simulink model "DYC0928"  (R2022b)
settings: Solver=VariableStepAuto  StartTime=0.0  StopTime=40  RelTol=1e-3
values from neighbouring files (symbols this model uses):
  Caf = 460    [trqvparameter.m]
  Car = 440    [trqvparameter.m]
  dwf = 1.2    [trqvparameter.m]
  dwr = 1.2    [trqvparameter.m]
  h = 0.29    [trqvparameter.m]
  i1 = 11.4    [trqvparameter.m]
  i2 = 3.4    [trqvparameter.m]
  Iz = 105    [trqvparameter.m]
  Kc = 10    [trqvparameter.m]
  Ki = 20    [trqvparameter.m]
  Kp = 30    [trqvparameter.m]
  lf = 0.761    [trqvparameter.m]
  lr = 0.831    [trqvparameter.m]
  m = 340    [trqvparameter.m]
  Rt = 0.2    [trqvparameter.m]
libraries: simulink x22, Solver_SF x1
settings Model: Creator=12045  LastModifiedBy=12045
settings OptimizationCC: DefaultParameterBehavior=Inlined  EnhancedBackFolding=on  PassReuseOutputArgsAs=Individual arguments  ZeroExternalMemoryAtStartup=off  ZeroInternalMemoryAtStartup=off  OptimizeBlockOrder=speed  DifferentSizesBufferReuse=on  OptimizationCustomize=off  EfficientTunableParamExpr=on
settings DebuggingCC: ParameterPrecisionLossMsg=none  ParameterTunabilityLossMsg=error
settings SFSimCC: MATLABDynamicMemAlloc=off
settings RTWCC: Description=Embedded Coder  SystemTargetFile=ert.tlc  TemplateMakefile=ert_default_tmf
settings CodeAppCC: ForceParamTrailComments=on  IgnoreCustomStorageClasses=off  OperatorAnnotations=on  SimulinkDataObjDesc=on  SFDataObjDesc=on  InsertBlockDesc=on
settings ERTTargetCC: TargetLangStandard=C99 (ISO)  GenerateSampleERTMain=on  InlinedParameterPlacement=NonHierarchical  ERTCustomFileTemplate=example_file_process.tlc

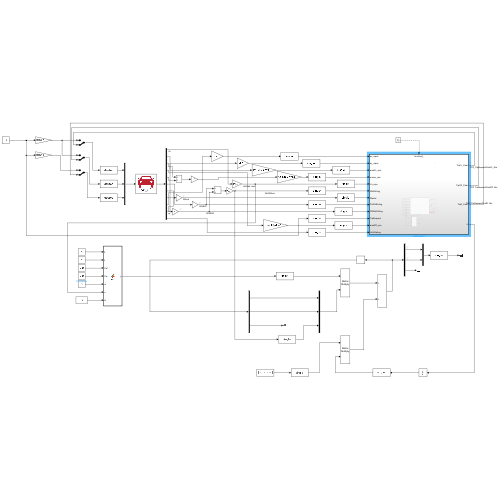
[thumbnail: Simulink's stored preview of the top-level diagram]
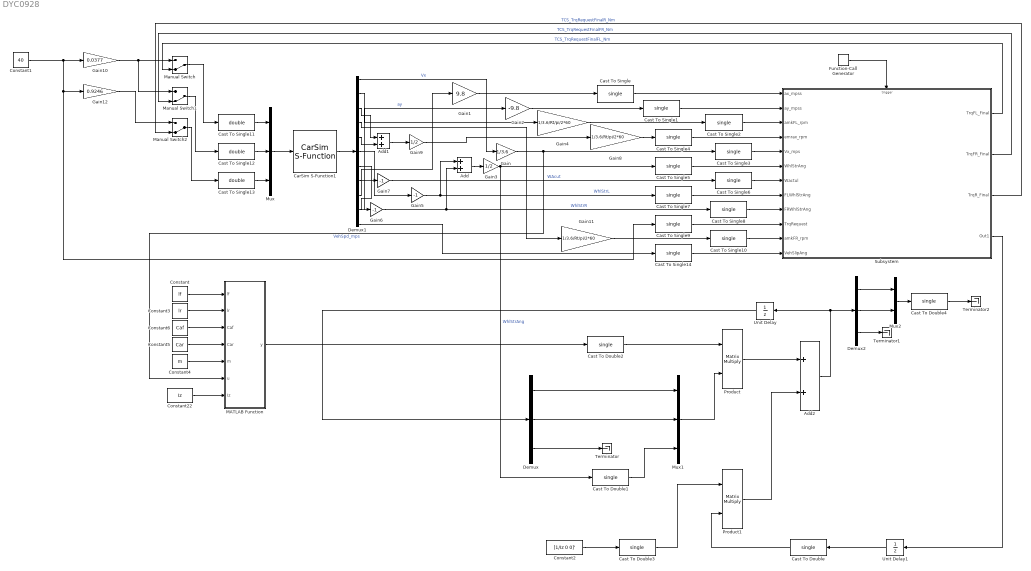
== system DYC0928 ==
  Add : Sum
  Add1 : Sum
  Add2 : Sum
  CarSim S-Function1 : Solver_SF/CarSim S-Function  Priority=1  SIMFILE=simfile.sim  Run_RTs=off  vs_state_ind=Run  StopMode_ind=Vehicle Model
  Cast To Double{,1..4} (5 alike) : DataTypeConversion  OutDataTypeStr=single  SaturateOnIntegerOverflow=off  RndMeth=Floor
  Cast To Single{,1..10,14} (12 alike) : DataTypeConversion  OutDataTypeStr=single  SaturateOnIntegerOverflow=off  RndMeth=Floor
  Cast To Single11 : DataTypeConversion  OutDataTypeStr=double  SaturateOnIntegerOverflow=off  RndMeth=Floor
  Cast To Single12 : DataTypeConversion  OutDataTypeStr=double  SaturateOnIntegerOverflow=off  RndMeth=Floor
  Cast To Single13 : DataTypeConversion  OutDataTypeStr=double  SaturateOnIntegerOverflow=off  RndMeth=Floor
  Constant : Constant  Value=lf
  Constant1 : Constant  Value=40
  Constant2 : Constant  Value=[1/Iz 0 0]'
  Constant22 : Constant  Value=Iz
  Constant3 : Constant  Value=lr
  Constant4 : Constant  Value=m
  Constant5 : Constant  Value=Car
  Constant6 : Constant  Value=Caf
  Demux : Demux  Outputs=3
  Demux1 : Demux  Outputs=11
  Demux2 : Demux  Outputs=3
  Function-Call Generator : simulink/Ports & Subsystems/Function-Call Generator  sample_time=0.01  numberOfIterations=1  DisallowWideOutput=off
  Gain : Gain  Gain=1/3.6
  Gain1 : Gain  Gain=9.8
  Gain10 : Gain  Gain=0.0377
  Gain11 : Gain  Gain=1/3.6/Rt/pi/2*60
  Gain12 : Gain  Gain=0.9246
  Gain2 : Gain  Gain=-9.8
  Gain3 : Gain  Gain=1/2
  Gain4 : Gain  Gain=1/3.6/Rt/pi/2*60
  Gain5 : Gain  Gain=-1
  Gain6 : Gain  Gain=-1
  Gain7 : Gain  Gain=-1
  Gain8 : Gain  Gain=1/3.6/Rt/pi/2*60
  Gain9 : Gain  Gain=1/2
  MATLAB Function : MATLAB Function  TreatAsAtomicUnit=on
  Manual Switch : ManualSwitch  CurrentSetting=0
  Manual Switch1 : ManualSwitch  CurrentSetting=0
  Manual Switch2 : ManualSwitch  CurrentSetting=0
  Mux : Mux  Inputs=3
  Mux1 : Mux  Inputs=3
  Mux2 : Mux  Inputs=2
  Product : Product  Multiplication=Matrix(*)
  Product1 : Product  Multiplication=Matrix(*)
  Subsystem : Subsystem
  Terminator : Terminator
  Terminator1 : Terminator
  Terminator2 : Terminator
  Unit Delay : UnitDelay  SampleTime=-1  HasFrameUpgradeWarning=on
  Unit Delay1 : UnitDelay  SampleTime=-1  HasFrameUpgradeWarning=on
  wires:
  Demux1/8 -> Gain1/1
  Gain2/1 -> Cast To Single1/1
  Gain4/1 -> Cast To Single2/1
  Gain8/1 -> Cast To Single4/1
  Gain3/1 -> Cast To Double1/1, Cast To Single5/1  "WhlStrAng"
  Constant1/1 -> Cast To Single9/1, Gain12/1, Gain10/1
  Function-Call Generator/1 -> Subsystem/Trigger
  Demux1/9 -> Gain7/1
  Demux1/10 -> Gain2/1  "ay"
  Mux/1 -> CarSim S-Function1/1
  Demux1/5 -> Add1/2
  Demux1/3 -> Add1/1
  Add1/1 -> Gain9/1
  Demux1/6 -> Gain5/1
  Demux1/7 -> Gain6/1
  Demux1/1 -> Gain/1  "Vx"
  CarSim S-Function1/1 -> Demux1/1
  Gain/1 -> MATLAB Function/6(u), Cast To Single3/1  "VehSpd_mps"
  Gain11/1 -> Cast To Single10/1
  Gain7/1 -> Cast To Single6/1  "WAcut"
  Gain1/1 -> Cast To Single/1
  Gain5/1 -> Add/1, Cast To Single7/1  "WhlStrL"
  Gain6/1 -> Add/2, Cast To Single8/1  "WhlStrR"
  Add/1 -> Gain3/1
  Demux1/4 -> Gain11/1
  Gain9/1 -> Gain8/1
  Demux1/2 -> Gain4/1
  Cast To Single/1 -> Subsystem/1(ax_mpss)
  Cast To Single1/1 -> Subsystem/2(ay_mpss)
  Cast To Single2/1 -> Subsystem/3(amkFL_rpm)
  Cast To Single3/1 -> Subsystem/5(Vx_mps)
  Cast To Single4/1 -> Subsystem/4(emrax_rpm)
  Cast To Single5/1 -> Subsystem/6(WhlStrAng)
  Cast To Single6/1 -> Subsystem/7(Wactul)
  Cast To Single7/1 -> Subsystem/8(FLWhlStrAng)
  Cast To Single8/1 -> Subsystem/9(FRWhlStrAng)
  Cast To Single9/1 -> Subsystem/10(TrqRequest)
  Cast To Single10/1 -> Subsystem/11(amkFR_rpm)
  Subsystem/3(TrqR_Final) -> Manual Switch2/2  "TCS_TrqRequestFinalR_Nm"
  Cast To Single11/1 -> Mux/1
  Cast To Single12/1 -> Mux/2
  Cast To Single13/1 -> Mux/3
  Subsystem/1(TrqFL_Final) -> Manual Switch/2  "TCS_TrqRequestFinalFL_Nm"
  Subsystem/2(TrqFR_Final) -> Manual Switch1/2  "TCS_TrqRequestFinalFR_Nm"
  Gain10/1 -> Manual Switch1/1, Manual Switch/1
  Manual Switch/1 -> Cast To Single11/1
  Manual Switch1/1 -> Cast To Single12/1
  Manual Switch2/1 -> Cast To Single13/1
  Gain12/1 -> Manual Switch2/1
  Demux1/11 -> Cast To Single14/1
  Cast To Single14/1 -> Subsystem/12(VehSlipAng)
  MATLAB Function/1(y) -> Cast To Double2/1
  Product/1 -> Add2/1
  Product1/1 -> Add2/2
  Constant2/1 -> Cast To Double3/1
  Subsystem/4(Out1) -> Unit Delay1/1
  Add2/1 -> Unit Delay/1, Demux2/1
  Unit Delay/1 -> Demux/1
  Mux1/1 -> Product/2
  Demux/1 -> Mux1/1
  Demux/2 -> Mux1/2
  Demux/3 -> Terminator/1
  Demux2/3 -> Terminator1/1
  Demux2/1 -> Mux2/1
  Demux2/2 -> Mux2/2
  Mux2/1 -> Cast To Double4/1
  Cast To Double/1 -> Product1/2
  Cast To Double1/1 -> Mux1/3
  Cast To Double2/1 -> Product/1
  Cast To Double3/1 -> Product1/1
  Cast To Double4/1 -> Terminator2/1
  Unit Delay1/1 -> Cast To Double/1
  Constant/1 -> MATLAB Function/1(lf)
  Constant3/1 -> MATLAB Function/2(lr)
  Constant6/1 -> MATLAB Function/3(Caf)
  Constant5/1 -> MATLAB Function/4(Car)
  Constant4/1 -> MATLAB Function/5(m)
  Constant22/1 -> MATLAB Function/7(Iz)

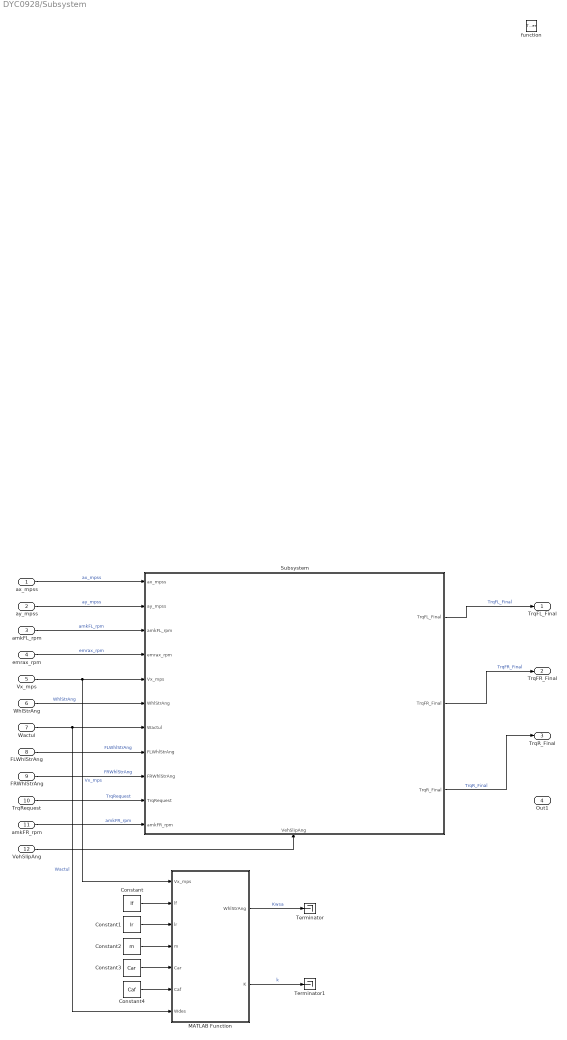
== system DYC0928/Subsystem ==
  ax_mpss : Inport
  ay_mpss : Inport  Port=2
  amkFL_rpm : Inport  Port=3
  emrax_rpm : Inport  Port=4
  Vx_mps : Inport  Port=5
  WhlStrAng : Inport  Port=6
  Wactul : Inport  Port=7
  FLWhlStrAng : Inport  Port=8
  FRWhlStrAng : Inport  Port=9
  TrqRequest : Inport  Port=10
  amkFR_rpm : Inport  Port=11
  VehSlipAng : Inport  Port=12
  function : TriggerPort  TriggerType=function-call  VariantControl=(inherit)
  Constant : Constant  Value=lf
  Constant1 : Constant  Value=lr
  Constant2 : Constant  Value=m
  Constant3 : Constant  Value=Car
  Constant4 : Constant  Value=Caf
  MATLAB Function : MATLAB Function  TreatAsAtomicUnit=on
  Subsystem : Subsystem
      settings: PortSchema="{\"entries\":[{\"content\":{\"sides\":[{\"content\":{\"connectorIds\":[\"In1\",\"In2\",\"In3\",\"In4\",\"In5\",\"In6\",\"In7\",\"In8\",\"In9\",\"In10\",\"In11\"]},\"type\":\"ConnectorPlacement.EquallySpacedRectSide\",\"uuid\":\"30ab71fb-d0f0-4095-97bb-bc920e154d4d\"},{\"content\":{\"connectorIds\":[\"Out1\",\"Out2\",\"Out3\"],\"side\":\"RIGHT\"},\"type\":\"ConnectorPlacement.EquallySpacedRectSide\",\"uuid\":\"88d0ca7e-fcea-4ec5-be14-2202af0b8b3f\"},{\"content\":{\"connectorIds\":[],\"side\":\"TOP\"},\"type\":\"ConnectorPlacement.EquallySpacedRectSide\",\"uuid\":\"a706d727-4e64-4be2-ad6e-9ac0966c97d4\"},{\"content\":{\"connectorIds\":[\"In12\"],\"side\":\"BOTTOM\"},\"type\":\"ConnectorPlacement.EquallySpacedRectSide\",\"uuid\":\"bad9005c-d910-4e7b-8a9f-d8b066b3db55\"}]},\"type\":\"ConnectorPlacement.EquallySpacedConnector\",\"uuid\":\"00d2e7d0-f9cc-4fcc-afd3-87106d3f46b0\"}],\"packageUris\":[\"http://schema.mathworks.com/mf0/Connector/R2020b\"],\"version\":\"1.0\"}"
  Terminator : Terminator
  Terminator1 : Terminator
  TrqFL_Final : Outport
  TrqFR_Final : Outport  Port=2
  TrqR_Final : Outport  Port=3
  Out1 : Outport  Port=4
  wires:
  ax_mpss/1 -> Subsystem/1(ax_mpss)  "ax_mpss"
  ay_mpss/1 -> Subsystem/2(ay_mpss)  "ay_mpss"
  amkFL_rpm/1 -> Subsystem/3(amkFL_rpm)  "amkFL_rpm"
  emrax_rpm/1 -> Subsystem/4(emrax_rpm)  "emrax_rpm"
  Vx_mps/1 -> MATLAB Function/1(Vx_mps), Subsystem/5(Vx_mps)  "Vx_mps"
  WhlStrAng/1 -> Subsystem/6(WhlStrAng)  "WhlStrAng"
  Wactul/1 -> MATLAB Function/7(Wdes), Subsystem/7(Wactul)  "Wactul"
  FLWhlStrAng/1 -> Subsystem/8(FLWhlStrAng)  "FLWhlStrAng"
  FRWhlStrAng/1 -> Subsystem/9(FRWhlStrAng)  "FRWhlStrAng"
  TrqRequest/1 -> Subsystem/10(TrqRequest)  "TrqRequest"
  amkFR_rpm/1 -> Subsystem/11(amkFR_rpm)  "amkFR_rpm"
  Subsystem/1(TrqFL_Final) -> TrqFL_Final/1  "TrqFL_Final"
  Subsystem/2(TrqFR_Final) -> TrqFR_Final/1  "TrqFR_Final"
  Subsystem/3(TrqR_Final) -> TrqR_Final/1  "TrqR_Final"
  Constant/1 -> MATLAB Function/2(lf)
  Constant1/1 -> MATLAB Function/3(lr)
  Constant2/1 -> MATLAB Function/4(m)
  Constant3/1 -> MATLAB Function/5(Car)
  Constant4/1 -> MATLAB Function/6(Caf)
  MATLAB Function/1(WhlStrAng) -> Terminator/1  "Kwsa"
  MATLAB Function/2(K) -> Terminator1/1  "k"
  VehSlipAng/1 -> Subsystem/12(VehSlipAng)
  ? -> Out1/1

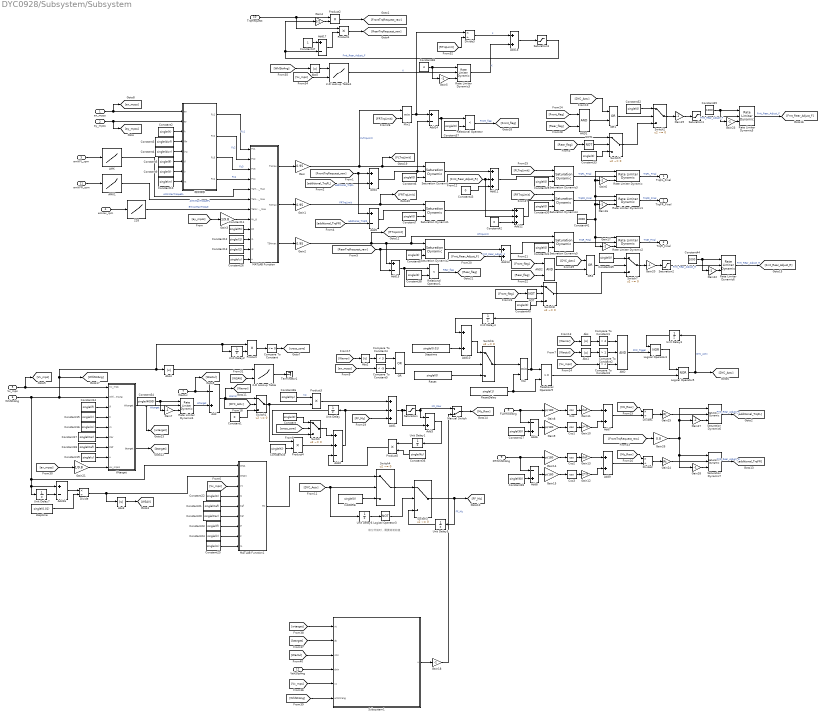
== system DYC0928/Subsystem/Subsystem ==
  note: 积分开始时，需要给初始值
  ax_mpss : Inport
  ay_mpss : Inport  Port=2
  amkFL_rpm : Inport  Port=3
  emrax_rpm : Inport  Port=4
  Vx_mps : Inport  Port=5
  WhlStrAng : Inport  Port=6
  Wactul : Inport  Port=7
  FLWhlStrAng : Inport  Port=8
  FRWhlStrAng : Inport  Port=9
  TrqRequest : Inport  Port=10
  amkFR_rpm : Inport  Port=11
  VehSlipAng : Inport  Port=12
  2-D Lookup Table : Lookup_n-D  BreakpointsForDimension1=[0 5 20 25]  BreakpointsForDimension2=[20 40 60]  Table=[3 5 8;5 8 10;6 10 13;8 12 14]  InternalRulePriority=Speed  RndMeth=Simplest
      settings: InputPortMap=u0,u1
  2-D Lookup Table1 : Lookup_n-D  BreakpointsForDimension1=[0;5;20;25;30]  BreakpointsForDimension2=[0;5;8;10;20;40;60]  Table=[0 0 0 0 0 0 0;0 0.3 0.45 0.5 0.53 0.55 0.58;0 0.4 0.55 0.56 0.58 0.62 0.65;0 0.55 0.7 0.72 0.78 0.81 0.83;0 0.6 0.8 0.82 0.86 0.89 0.9]  InternalRulePriority=Speed  RndMeth=Simplest
      settings: InputPortMap=u0,u1
  228 : Lookup_n-D  NumberOfTableDimensions=1  BreakpointsForDimension1=[200;400;600;800;1000;1200;1400;1600;1800;2000;2200;2400;2600;2800;3000;3200;3400;3600;3800;4000;4200;4400;4600;4800;5000;5200;5400]  BreakpointsForDimension2=[1:3]  Table=[229.85;229.85;229.85;229.85;229.85;229.85;229.85;229.85;229.85;229.85;229.85;229.85;229.46;229.16;228.86;228.86;228.86;228.86;228.86;227.86;227.86;226.87;225.86;224.86;220.86;218.87;215.87]  InternalRulePriority=Speed  RndMeth=Simplest
  AMK : Lookup_n-D  NumberOfTableDimensions=1  BreakpointsForDimension1=[0;1000;2000;3000;4000;5000;6000;7000;8000;9000;10000;11000;12000;13000;14000;15000;16000;17000;18000;19000]  BreakpointsForDimension2=[1:3]  Table=[21;21;21;21;21;21;21;21;21;21;21;21;21;21;20;17.5;15;12.5;8;0]  InternalRulePriority=Speed  RndMeth=Simplest
  AMK1 : Lookup_n-D  NumberOfTableDimensions=1  BreakpointsForDimension1=[0;1000;2000;3000;4000;5000;6000;7000;8000;9000;10000;11000;12000;13000;14000;15000;16000;17000;18000;19000]  BreakpointsForDimension2=[1:3]  Table=[21;21;21;21;21;21;21;21;21;21;21;21;21;21;20;17.5;15;12.5;8;0]  InternalRulePriority=Speed  RndMeth=Simplest
  AND : Logic  Inputs=3  AllPortsSameDT=off  OutDataTypeStr=boolean
  AND1 : Logic  AllPortsSameDT=off  OutDataTypeStr=boolean
  AND2 : Logic  AllPortsSameDT=off  OutDataTypeStr=boolean
  Abs{,1..5} (6 alike) : Abs  SaturateOnIntegerOverflow=off
  Add{,3,6,8} (4 alike) : Sum  Inputs=-+
  Add1 : Sum  Inputs=+++
  Add{4,7,9..10,13,18} (6 alike) : Sum
  Add11 : Sum  Inputs=+++
  Add12 : Sum  Inputs=+++
  Add{5,14..17} (5 alike) : Sum  Inputs=+-
  Add2 : Sum  Inputs=++-
  Compare To Constant : simulink/Logic and Bit Operations/Compare To Constant  relop=<=  const=0  OutDataTypeStr=boolean
  Compare To Constant1 : simulink/Logic and Bit Operations/Compare To Constant  relop=>  const=4  OutDataTypeStr=boolean
  Compare To Constant2 : simulink/Logic and Bit Operations/Compare To Constant  relop=>  const=1  OutDataTypeStr=boolean
  Compare To Constant3 : simulink/Logic and Bit Operations/Compare To Constant  relop=>  const=2  OutDataTypeStr=boolean
  Compare To Constant4 : simulink/Logic and Bit Operations/Compare To Constant  relop=<  const=3  OutDataTypeStr=boolean
  Compare To Constant5 : simulink/Logic and Bit Operations/Compare To Constant  relop=<  const=-5  OutDataTypeStr=boolean
  Constant{,6..8,29..33,37..40} (13 alike) : Constant  Value=single(0)
  Constant1 : Constant  Value=0
  Constant10 : Constant  Value=single(m)
  Constant11 : Constant  Value=single(Rt)
  Constant12 : Constant  Value=single(i1)
  Constant13 : Constant  Value=single(i2)
  Constant14 : Constant  Value=single(lf)
  Constant15 : Constant  Value=single(lr)
  Constant16 : Constant  Value=single(m)
  Constant17 : Constant  Value=single(Car)
  Constant18 : Constant  Value=single(Caf)
  Constant19 : Constant  Value=single(u)
  Constant2 : Constant  Value=single(h)
  Constant20 : Constant  Value=single(Car)
  Constant21 : Constant  Value=single(Caf)
  Constant22 : Constant  Value=single(Iz)
  Constant23 : Constant  Value=single(lf)
  Constant24 : Constant  Value=single(lr)
  Constant25 : Constant  Value=single(m)
  Constant26 : Constant  Value=single(u)
  Constant27 : Constant  Value=single(90)
  Constant28 : Constant  Value=single(90)
  Constant3 : Constant  Value=single(dwf)
  Constant34 : Constant  Value=single(4000)
  Constant35 : Constant  Value=single(Ki)
  Constant36 : Constant  Value=single(Kc)
  Constant4 : Constant  Value=single(dwr)
  Constant41 : Constant  Value=2000
  Constant42 : Constant  Value=0
  Constant43 : Constant  Value=0
  Constant44 : Constant  Value=1000
  Constant45 : Constant  Value=1000
  Constant46 : Constant  Value=single(Kp)
  Constant47 : Constant
  Constant48 : Constant  Value=4
  Constant5 : Constant  Value=single(lf)
  Constant9 : Constant  Value=single(lr)
  Cos{,1..3} (4 alike) : Trigonometry  Operator=cos
  Divide{,1..3} (4 alike) : Product  Inputs=*/
  Gain : Gain  Gain=0.95
  Gain1 : Gain  Gain=0.95
  Gain10 : Gain  Gain=2*lf
  Gain11 : Gain  Gain=dwf
  Gain12 : Gain  Gain=2*lf
  Gain13 : Gain  Gain=dwf
  Gain{8..9,14..15} (4 alike) : Gain  Gain=pi/180
  Gain{5..7,16..20,22..23,27..28} (12 alike) : Gain  Gain=-1
  Gain2 : Gain  Gain=0.95
  Gain21 : Gain  Gain=1/9.8
  Gain24 : Gain  Gain=Rt
  Gain25 : Gain  Gain=Rt
  Gain26 : Gain  Gain=0.8
  Gain3 : Gain  Gain=1/9.8
  Gain4 : Gain  Gain=1/2
  InitZORE : Constant  Value=single(0)
  Logical Operator3 : Logic  Operator=NOT  AllPortsSameDT=off  OutDataTypeStr=boolean
  Logical Operator4 : Logic  Operator=NOR  AllPortsSameDT=off  OutDataTypeStr=boolean
  Logical Operator5 : Logic  Operator=NOR  AllPortsSameDT=off  OutDataTypeStr=boolean
  MATLAB Function : MATLAB Function  TreatAsAtomicUnit=on
  MATLAB Function1 : MATLAB Function  TreatAsAtomicUnit=on
  Manual Switch : ManualSwitch  CurrentSetting=0
  Min : MinMax  Inputs=2
  Min1 : MinMax  Inputs=2
  NOT : Logic  Operator=NOT  AllPortsSameDT=off  OutDataTypeStr=boolean
  NOT1 : Logic  Operator=NOT  AllPortsSameDT=off  OutDataTypeStr=boolean
  OR : Logic  Operator=OR  AllPortsSameDT=off  OutDataTypeStr=boolean
  OR1 : Logic  Operator=OR  AllPortsSameDT=off  OutDataTypeStr=boolean
  OR2 : Logic  Operator=OR  AllPortsSameDT=off  OutDataTypeStr=boolean
  Product{,1..5} (6 alike) : Product
  Rate Limiter Dynamic{,1..6} (7 alike) : simulink/Discontinuities/Rate Limiter Dynamic
  Relational Operator : RelationalOperator  Operator=<  OutDataTypeStr=boolean  RndMeth=Simplest  InputSameDT=off
  Relational Operator1 : RelationalOperator  Operator=<  OutDataTypeStr=boolean  RndMeth=Simplest  InputSameDT=off
  Relational Operator9 : RelationalOperator  OutDataTypeStr=boolean  RndMeth=Simplest  InputSameDT=off
  Reset : Constant  Value=single(0)
  ResetDelay : Constant  Value=single(1)
  Saturation : Saturate  UpperLimit=5000  LowerLimit=-5000
  Saturation Dynamic{,1..7} (8 alike) : simulink/Discontinuities/Saturation Dynamic  OutMin=[]  OutMax=[]  OutDataTypeStr=Inherit: Same as second input  OutDataType=fixdt(1, 16)  OutScaling=2^-10  DoSatur=off
  Saturation1 : Saturate  UpperLimit=100  LowerLimit=0
  Saturation2 : Saturate  UpperLimit=100  LowerLimit=0
  Saturation3 : Saturate  UpperLimit=0.7  LowerLimit=0.1
  Steptime : Constant  Value=single(0.01)
  Subsystem1 : Subsystem
  Switch{,1..8} (9 alike) : Switch  Criteria=u2 ~= 0  SaturateOnIntegerOverflow=off  InputSameDT=off
  Terminator1 : Terminator
  Unit Delay{,1..7} (8 alike) : UnitDelay  SampleTime=-1  HasFrameUpgradeWarning=on
  Wtarget : MATLAB Function  TreatAsAtomicUnit=on
  steptime : Constant  Value=single(0.01)
  载荷转移 : MATLAB Function  TreatAsAtomicUnit=on
  TrqFL_Final : Outport
  TrqFR_Final : Outport  Port=2
  TrqR_Final : Outport  Port=3
  wires:
  2-D Lookup Table1/1 -> Rate Limiter Dynamic3/2  "K"
  [ay_mpss] -> Gain3/1
  载荷转移/4(Fz4) -> MATLAB Function/4(Fz4)  "Fz4"
  MATLAB Function/3(T34max) -> Gain2/1
  TrqRequest/1 -> Product2/1, Product1/1
  Gain/1 -> Min1/1, [FLTrqLimit], Saturation Dynamic/1  "FLTrqLimit"
  Constant33/1 -> Switch5/3
  Constant23/1 -> MATLAB Function1/7(lf)
  Gain16/1 -> Rate Limiter Dynamic1/3
  Gain11/1 -> Add7/1
  [FRTrqLimit] -> Min1/2
  载荷转移/1(Fz1) -> MATLAB Function/1(Fz1)  "Fz1"
  OR/1 -> Switch6/2
  Unit Delay5/1 -> Switch3/3
  OR1/1 -> Switch2/2
  Gain27/1 -> Saturation Dynamic6/3
  AND1/1 -> OR1/2
  Steptime/1 -> Add10/2
  FLWhlStrAng/1 -> Add6/1, Gain8/1
  Add14/1 -> Relational Operator/1, Switch5/1
  Constant35/1 -> Product4/2
  Constant30/1 -> Saturation Dynamic4/3
  Wactul/1 -> Add/1, [Wactul]
  Add13/1 -> Saturation Dynamic5/2
  Unit Delay/1 -> Switch/3
  Constant3/1 -> 载荷转移/4(lfw)
  Unit Delay6/1 -> Logical Operator3/1
  Divide3/1 -> Add18/1  "k"
  [RearTrqRequest_raw] -> Saturation Dynamic2/2, Add15/2
  [Front_flag] -> NOT/1
  [Vx_mps] -> MATLAB Function1/3(Vx)
  Gain26/1 -> Saturation Dynamic6/1, Gain27/1, Gain28/1, Saturation Dynamic7/1
  Rate Limiter Dynamic6/1 -> [Frnt_Rear_Adjust_R]  "Frnt_Rear_Adjust_R"
  [ax_mpss] -> Gain21/1
  Constant16/1 -> Wtarget/5(m)
  Constant1/1 -> Switch1/3
  Gain17/1 -> Rate Limiter Dynamic2/3
  Saturation Dynamic5/1 -> Rate Limiter Dynamic2/2  "TrqR_Final"
  Divide2/1 -> Gain24/1
  AMK1/1 -> MATLAB Function/6(TamkFR_max)  "AMKMaxTroqueFL"
  AMK/1 -> MATLAB Function/5(TamkFL_max)  "AMKMaxTroqueFL"
  2-D Lookup Table/1 -> Terminator1/1
  Constant8/1 -> Saturation Dynamic2/3
  Constant15/1 -> Wtarget/4(lr)
  ay_mpss/1 -> 载荷转移/2(ay), [ay_mpss]
  Constant45/1 -> Gain23/1, Rate Limiter Dynamic5/1
  Gain6/1 -> Rate Limiter Dynamic/3
  Gain7/1 -> Rate Limiter Dynamic4/3
  Gain20/1 -> Saturation2/1
  Add11/1 -> Saturation Dynamic3/2
  Constant10/1 -> 载荷转移/8(m)
  Gain19/1 -> Saturation1/1
  载荷转移/3(Fz3) -> MATLAB Function/3(Fz3)  "Fz3"
  Saturation Dynamic1/1 -> Add12/1
  Gain2/1 -> [RTrqLimit], Add15/1, Saturation Dynamic5/1, Saturation Dynamic2/1  "RTrqLimit"
  228/1 -> MATLAB Function/7(Temrax_max)  "EmraxMaxTroque"
  [WSAV] -> 2-D Lookup Table/2
  Gain23/1 -> Rate Limiter Dynamic5/3
  Add1/1 -> Saturation/1, Add3/2
  Add7/1 -> Divide1/2
  steptime/1 -> Divide/2
  Add/1 -> [Werror], Switch1/1  "Werror"
  Add17/1 -> Product1/2
  Wtarget/1(Wtarget) -> Rate Limiter Dynamic4/2, [wtarget]  "Wtarget"
  Constant6/1 -> Saturation Dynamic/3
  Unit Delay1/1 -> Product5/1
  emrax_rpm/1 -> 228/1
  Rate Limiter Dynamic4/1 -> Add/2  "Wtarget"
  Constant11/1 -> MATLAB Function/9(Rt)
  Reset/1 -> Switch6/3
  Saturation2/1 -> Rate Limiter Dynamic6/2  "Frnt_Rear_Adjust_R"
  OR2/1 -> Switch7/2
  Abs/1 -> Compare To Constant1/1
  [Front_flag] -> AND1/1
  Constant41/1 -> Rate Limiter Dynamic/1, Gain6/1, Rate Limiter Dynamic1/1, Gain16/1, Gain17/1, Rate Limiter Dynamic2/1
  ax_mpss/1 -> [ax_mpss], 载荷转移/1(ax)
  Saturation Dynamic2/1 -> Add13/1
  FRWhlStrAng/1 -> Gain14/1, Add8/1
  Cos1/1 -> Gain10/1
  Min1/1 -> Divide3/1, Add14/1
  Unit Delay2/1 -> Product/2
  Compare To Constant/1 -> [cross_zore]
  AND2/1 -> OR2/2
  Saturation1/1 -> Rate Limiter Dynamic5/2  "Frnt_Rear_Adjust_F"
  Relational Operator1/1 -> [Rear_flag]  "Rear_flag"
  Product5/1 -> Add2/3
  Constant44/1 -> Gain22/1, Rate Limiter Dynamic6/1
  Constant19/1 -> Wtarget/8(u)
  Saturation Dynamic3/1 -> Rate Limiter Dynamic/2  "TrqFL_Final"
  Constant25/1 -> MATLAB Function1/9(m)
  [Front_flag] -> AND2/1
  [DYC_Actv] -> OR1/1
  Gain3/1 -> MATLAB Function/8(ay_g)
  Product4/1 -> Add2/2
  Cos2/1 -> Gain13/1
  Logical Operator3/1 -> Switch3/2
  Switch/1 -> Add2/1
  Switch8/1 -> Switch7/3
  Constant36/1 -> Product5/2
  [DYC_Actv] -> Switch1/2
  WhlStrAng/1 -> Product/1, Unit Delay2/1, Abs4/1, [WhlStrAng], Wtarget/2(WhlStrAng), MATLAB Function1/1(WSA), Add16/1, Unit Delay7/1
  Constant27/1 -> Add6/2
  AND/1 -> Logical Operator4/2  "DYC_Tigger"
  [Mz_Raw] -> Divide2/1
  Gain10/1 -> Add7/2
  Constant20/1 -> MATLAB Function1/6(Car)
  Gain28/1 -> Saturation Dynamic7/3
  [Rear_flag] -> AND2/2
  Saturation/1 -> Manual Switch/1, Add3/1  "Mz_Raw"
  Constant22/1 -> MATLAB Function1/4(Iz)
  Wtarget/2(btarget) -> [btarget]
  Constant46/1 -> Product3/1  "Kp"
  ResetDelay/1 -> Relational Operator9/2, Min/2
  Constant26/1 -> MATLAB Function/12(u)
  Gain13/1 -> Add9/1
  Constant9/1 -> 载荷转移/7(lr)
  Constant40/1 -> Switch8/3
  Constant2/1 -> 载荷转移/3(h)
  [Werror] -> Abs/1
  Compare To Constant1/1 -> AND/1
  amkFR_rpm/1 -> AMK1/1
  MATLAB Function/2(T2max) -> Gain1/1
  Constant34/1 -> Rate Limiter Dynamic4/1, Gain7/1
  Product2/1 -> [FrontTrqRequest_raw]
  Divide/1 -> Abs3/1, MATLAB Function1/2(WSAV)
  Constant/1 -> Switch/1
  Rate Limiter Dynamic1/1 -> TrqFR_Final/1  "TrqFR_Final"
  Switch1/1 -> Product4/1, Product3/2
  Logical Operator5/1 -> [DYC_Actv], Unit Delay3/1  "DYC_Actv"
  Rate Limiter Dynamic/1 -> TrqFL_Final/1  "TrqFL_Final"
  Add8/1 -> Gain15/1
  Min/1 -> Unit Delay4/1, Relational Operator9/1
  Constant47/1 -> Add17/1
  Constant48/1 -> Gain5/1, Rate Limiter Dynamic3/1
  Unit Delay7/1 -> Add16/2
  MATLAB Function/1(T1max) -> Gain/1
  Switch2/1 -> Gain19/1
  Gain8/1 -> Cos/1
  InitZORE/1 -> Switch4/3
  Product1/1 -> [RearTrqRequest_raw]
  Add4/1 -> Add14/2, Saturation Dynamic/2
  Gain14/1 -> Cos2/1
  Relational Operator9/1 -> Logical Operator5/2
  Add3/1 -> Unit Delay1/1
  [Frnt_Rear_Adjust_F] -> Add13/2  "Frnt_Rear_Adjust_F"
  Gain12/1 -> Add9/2
  Add10/1 -> Switch6/1
  [Wactul] -> Abs1/1
  Abs1/1 -> Compare To Constant2/1
  Constant24/1 -> MATLAB Function1/8(lr)
  Compare To Constant5/1 -> OR/2
  Switch3/1 -> [FF_Mz], Unit Delay5/1  "FF_Mz"
  Switch6/1 -> Min/1
  Rate Limiter Dynamic2/1 -> TrqR_Final/1  "TrqR_Final"
  Constant39/1 -> Switch7/1
  [Werror] -> Abs2/1
  [DYC_Actv] -> Unit Delay6/1, Switch4/2
  Gain1/1 -> [FRTrqLimit], Saturation Dynamic1/1  "FRTrqLimit"
  Saturation Dynamic7/1 -> [additional_TrqFR]  "Frnt_Rear_Adjust_R"
  Gain25/1 -> Saturation Dynamic6/2
  Divide1/1 -> Gain25/1
  Rate Limiter Dynamic5/1 -> [Frnt_Rear_Adjust_F]  "Frnt_Rear_Adjust_F"
  Constant5/1 -> 载荷转移/6(lf)
  Add5/1 -> Saturation Dynamic1/2
  Add15/1 -> Switch8/1, Relational Operator1/1
  Constant28/1 -> Add8/2
  [FrontTrqRequest_raw] -> Gain26/1
  Switch7/1 -> Gain20/1
  Compare To Constant2/1 -> AND/2
  Add9/1 -> Divide2/2
  Gain5/1 -> Rate Limiter Dynamic3/3
  Gain15/1 -> Cos3/1
  Add2/1 -> Add1/2, Unit Delay/1
  amkFL_rpm/1 -> AMK/1
  [additional_TrqFR] -> Add5/2  "additional_TrqFR"
  Constant31/1 -> Saturation Dynamic5/3
  Unit Delay4/1 -> Add10/1
  Add6/1 -> Gain9/1
  [ax_mpss] -> Compare To Constant5/1
  Abs5/1 -> 2-D Lookup Table1/1
  Logical Operator4/1 -> Logical Operator5/1
  Vx_mps/1 -> Wtarget/1(Vx_mps), [Vx_mps]
  Cos/1 -> Gain11/1
  Unit Delay3/1 -> Logical Operator4/1
  Saturation Dynamic/1 -> Add11/1
  Gain9/1 -> Cos1/1
  [Frnt_Rear_Adjust_R] -> Add12/2, Add11/2
  [DYC_Actv] -> OR2/1
  [Mz_Raw] -> Divide1/1
  Saturation Dynamic4/1 -> Rate Limiter Dynamic1/2  "TrqFR_Final"
  Product/1 -> Compare To Constant/1
  Saturation Dynamic6/1 -> [additional_TrqFL]  "Frnt_Rear_Adjust_R"
  Constant29/1 -> Saturation Dynamic3/3
  [FLTrqLimit] -> Saturation Dynamic3/1
  MATLAB Function1/1(Mz) -> Switch4/1
  Constant12/1 -> MATLAB Function/10(i1)
  [FRTrqLimit] -> Saturation Dynamic4/1
  Constant14/1 -> Wtarget/3(lf)
  NOT1/1 -> Switch5/2
  Relational Operator/1 -> [Front_flag]  "Front_flag"
  Switch4/1 -> Switch3/1
  Constant38/1 -> Relational Operator1/2
  Constant7/1 -> Saturation Dynamic1/3
  [cross_zore] -> Switch/2
  Constant18/1 -> Wtarget/7(Caf)
  Constant37/1 -> Relational Operator/2
  [Vx_mps] -> Compare To Constant3/1
  Compare To Constant4/1 -> OR/1
  NOT/1 -> Switch8/2
  Add12/1 -> Saturation Dynamic4/2
  [additional_TrqFL] -> Add4/2  "additional_TrqFL"
  Constant4/1 -> 载荷转移/5(lrw)
  Saturation3/1 -> Gain4/1, Add17/2  "Frnt_Rear_Adjust_F"
  [Rear_flag] -> NOT1/1
  Add16/1 -> Divide/1
  Gain4/1 -> Product2/2
  [FrontTrqRequest_raw] -> Add5/1, Add4/1
  Switch5/1 -> Switch2/3
  Constant13/1 -> MATLAB Function/11(i2)
  [Rear_flag] -> AND1/2
  Gain22/1 -> Rate Limiter Dynamic6/3
  Abs3/1 -> [WSAV]
  Rate Limiter Dynamic3/1 -> Add18/2  "K"
  Abs4/1 -> 2-D Lookup Table/1
  Constant21/1 -> MATLAB Function1/5(Caf)
  [FF_Mz] -> Add1/3
  Constant32/1 -> Switch2/1
  Gain21/1 -> Wtarget/9(Ax_mpss)
  Product3/1 -> Add1/1
  Compare To Constant3/1 -> AND/3
  Constant42/1 -> Add12/3
  Abs2/1 -> Compare To Constant4/1
  Constant43/1 -> Add11/3
  [Vx_mps] -> 2-D Lookup Table1/2
  载荷转移/2(Fz2) -> MATLAB Function/2(Fz2)  "Fz2"
  Add18/1 -> Saturation3/1
  Cos3/1 -> Gain12/1
  Gain24/1 -> Saturation Dynamic7/2
  [WhlStrAng] -> Abs5/1
  Constant17/1 -> Wtarget/6(Car)
  [RTrqLimit] -> Divide3/2
  [Wactul] -> Subsystem1/3(xtin)
  [wtarget] -> Subsystem1/1(xt)
  Subsystem1/1(u) -> Gain18/1
  [btarget] -> Subsystem1/2(dt)
  [Vx_mps] -> Subsystem1/5(vx)
  [WhlStrAng] -> Subsystem1/6(whlstrang)
  VehSlipAng/1 -> Subsystem1/4(dxin)
  Gain18/1 -> Manual Switch/2
  Manual Switch/1 -> [Mz_Raw]

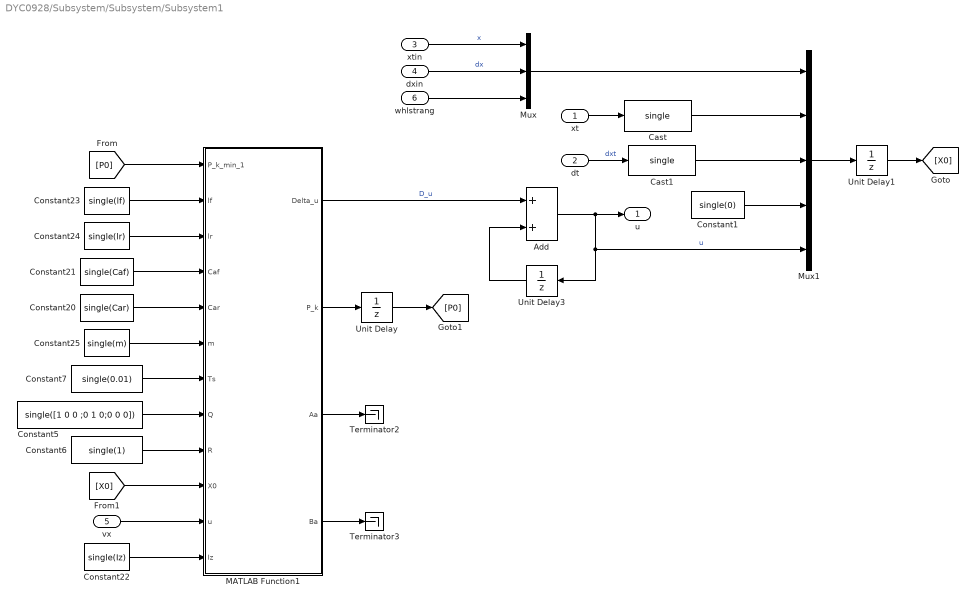
== system DYC0928/Subsystem/Subsystem/Subsystem1 ==
  xt : Inport
  dt : Inport  Port=2
  xtin : Inport  Port=3
  dxin : Inport  Port=4
  vx : Inport  Port=5
  whlstrang : Inport  Port=6
  Add : Sum
  Cast : DataTypeConversion  OutDataTypeStr=single  SaturateOnIntegerOverflow=off  RndMeth=Floor
  Cast1 : DataTypeConversion  OutDataTypeStr=single  SaturateOnIntegerOverflow=off  RndMeth=Floor
  Constant1 : Constant  Value=single(0)
  Constant20 : Constant  Value=single(Car)
  Constant21 : Constant  Value=single(Caf)
  Constant22 : Constant  Value=single(Iz)
  Constant23 : Constant  Value=single(lf)
  Constant24 : Constant  Value=single(lr)
  Constant25 : Constant  Value=single(m)
  Constant5 : Constant  Value=single([1 0 0 ;0 1 0;0 0 0])
  Constant6 : Constant  Value=single(1)
  Constant7 : Constant  Value=single(0.01)
  MATLAB Function1 : MATLAB Function  TreatAsAtomicUnit=on
  Mux : Mux  Inputs=3
  Mux1 : Mux  Inputs=5
  Terminator2 : Terminator
  Terminator3 : Terminator
  Unit Delay : UnitDelay  InitialCondition=[eye(3) -eye(3) zeros(3,1)]'*[100 0 0;0 1 0;0 0 0]*[eye(3) -eye(3) zeros(3,1)]  SampleTime=-1  HasFrameUpgradeWarning=on
  Unit Delay1 : UnitDelay  InitialCondition=[0 0 0 0 0 0 0]'  SampleTime=-1  HasFrameUpgradeWarning=on
  Unit Delay3 : UnitDelay  SampleTime=-1  HasFrameUpgradeWarning=on
  u : Outport
  wires:
  MATLAB Function1/4(Ba) -> Terminator3/1
  Add/1 -> u/1, Mux1/5, Unit Delay3/1  "u"
  xtin/1 -> Mux/1  "x"
  MATLAB Function1/1(Delta_u) -> Add/1  "D_u"
  xt/1 -> Cast/1
  dxin/1 -> Mux/2  "dx"
  Unit Delay3/1 -> Add/2
  MATLAB Function1/3(Aa) -> Terminator2/1
  Unit Delay1/1 -> [X0]
  [X0] -> MATLAB Function1/10(X0)
  Unit Delay/1 -> [P0]
  dt/1 -> Cast1/1  "dxt"
  Mux/1 -> Mux1/1
  Mux1/1 -> Unit Delay1/1
  Constant5/1 -> MATLAB Function1/8(Q)
  Cast/1 -> Mux1/2
  MATLAB Function1/2(P_k) -> Unit Delay/1
  Constant6/1 -> MATLAB Function1/9(R)
  [P0] -> MATLAB Function1/1(P_k_min_1)
  Constant25/1 -> MATLAB Function1/6(m)
  Constant7/1 -> MATLAB Function1/7(Ts)
  Constant21/1 -> MATLAB Function1/4(Caf)
  Constant20/1 -> MATLAB Function1/5(Car)
  Constant23/1 -> MATLAB Function1/2(lf)
  Constant24/1 -> MATLAB Function1/3(lr)
  vx/1 -> MATLAB Function1/11(u)
  Constant22/1 -> MATLAB Function1/12(Iz)
  Cast1/1 -> Mux1/3
  Constant1/1 -> Mux1/4
  whlstrang/1 -> Mux/3

== matlab function DYC0928/Subsystem/Subsystem/Subsystem1/MATLAB Function1 ==
  data: Delta_u output; P_k_min_1 input single; lf input; lr input single; Caf input; Car input; m input; Ts input; Q input; R input; P_k output single; X0 input single; Aa output; Ba output; u input; Iz input
function [Delta_u,P_k,Aa,Ba] = fcn(P_k_min_1,lf,lr,Caf,Car,m,Ts,Q,R,X0,u,Iz)
Aa_ = [(lf*lf*Caf+lr*lr*Car)/Iz/u (lf*Caf-lr*Car)/Iz -lf*Caf/Iz;((lf*Caf-lr*Car)/m/u/u)-1 (lf+lr)/m/u -Caf/m/u;0 0 0];
Ba_ = [1/Iz 0 0]';
AD = [0 1 0;0 0 0;0 0 0];
n = size (Aa_,1);
p = size(Ba_,2);
Ca =[eye(n) -eye(n) zeros(n,p)];
A = expm(Aa_*Ts);
B = pinv(Aa_)*(A-eye(n))*Ba_;
Ad = expm(AD*Ts);
Aa = [A zeros(n) B;zeros(n) Ad zeros(n,p);zeros(p,n) zeros(p,n) eye(p,p)];
Ba = [B;zeros(n,p);eye(p)];
Qa = transpose(Ca)*Q*Ca;
F_N_min_k = pinv(R+Ba'*P_k_min_1*Ba)*Ba'*P_k_min_1*Aa;
P_k = (Aa-Ba*F_N_min_k)'*P_k_min_1*(Aa-Ba*F_N_min_k)+(F_N_min_k)'*R*(F_N_min_k)+Qa;
Delta_u = -F_N_min_k*X0;

== matlab function DYC0928/MATLAB Function ==
  data: lf input; lr input; Caf input; Car input; m input; u input; y output; Iz input
function y = fcn(lf,lr,Caf,Car,m,u,Iz)

y = [(lf*lf*Caf+lr*lr*Car)/Iz/u (lf*Caf-lr*Car)/Iz -lf*Caf/Iz;((lf*Caf-lr*Car)/m/u/u)-1 (lf+lr)/m/u -Caf/m/u;0 0 0];

== matlab function DYC0928/Subsystem/Subsystem/Wtarget ==
  data: Vx_mps input size=1; Wtarget output size=1; WhlStrAng input size=1; btarget output; lf input; lr input; m input; Car input; Caf input; u input; Ax_mpss input
function [Wtarget,btarget] = fcn(Vx_mps,WhlStrAng,lf,lr,m,Car,Caf,u,Ax_mpss)
Wdes = Vx_mps*WhlStrAng/(lf+lr+(m*Vx_mps*Vx_mps*(lr*Car-lf*Caf)/Caf/Car/(lr+lf)/2));
Wu = 0.8*u*9.8/Ax_mpss;
temp = min(abs(Wu),abs(Wdes));
    Wtarget = 0.6*temp*sign(Wdes);
%     Wtarget = Wdes;

bdes = (lr-lf*m*Vx_mps*Vx_mps/Car/(lf+lr)/2)*WhlStrAng/(lr+lf+m*Vx_mps*Vx_mps*(lr*Car-lf*Caf)/Car/Caf/(lf+lr)/2);
bu = atan(0.02*u*9.8);
if abs(bdes)<=bu
btarget = bdes;
else
    btarget = bu*sign(bdes);
end

== matlab function DYC0928/Subsystem/Subsystem/MATLAB Function ==
  data: Fz1 input; T1max output; Fz2 input; Fz3 input; Fz4 input; T2max output; T34max output; TamkFL_max input; TamkFR_max input; Temrax_max input; ay_g input; Rt input; i1 input; i2 input; u input
function [T1max,T2max,T34max] = fcn(Fz1,Fz2,Fz3,Fz4, TamkFL_max,TamkFR_max, Temrax_max,ay_g,Rt,i1,i2,u)
g = 9.8;

Fx1 = sqrt(power(Fz1*u,2)-power(Fz1*ay_g/g,2));
Fx2 = sqrt(power(Fz2*u,2)-power(Fz2*ay_g/g,2));
Fx3 = sqrt(power(Fz3*u,2)-power(Fz3*ay_g/g,2));
Fx4 = sqrt(power(Fz4*u,2)-power(Fz4*ay_g/g,2));


T1max = min(Fx2*Rt/i1,TamkFR_max);
T2max = min(Fx1*Rt/i1,TamkFL_max);
T34max = min(min(Fx4,Fx3)*Rt/i2,Temrax_max);

== matlab function DYC0928/Subsystem/Subsystem/MATLAB Function1 ==
  data: WSA input; Mz output; WSAV input; Vx input; Iz input; Caf input; Car input; lf input; lr input; m input
function Mz = fcn(WSA,WSAV,Vx,Iz,Caf,Car,lf,lr,m)

Mz = ((((lf*lf*Caf+lr*lr*Car)/Iz/Vx)*(-Caf/m/Vx)-((lf*Caf-lr*Car)/m/Vx/Vx-1)*(-lf*Caf/Iz))*Iz*WSA-(-Caf/m/Vx)*Iz*WSAV)/((lf*Caf-lr*Car)/m/Vx/Vx-1)/100;

== matlab function DYC0928/Subsystem/MATLAB Function ==
  data: Vx_mps input; lf input; lr input; m input; Car input; Caf input; WhlStrAng output; Wdes input; K output
function [WhlStrAng,K] = fcn(Vx_mps,lf,lr,m,Car,Caf,Wdes)
WhlStrAng = Wdes/Vx_mps*(lf+lr+(m*Vx_mps*Vx_mps*(lr*Car-lf*Caf)/Caf/Car/(lr+lf)/2));
K = Vx_mps/(lf+lr+(m*Vx_mps*Vx_mps*(lr*Car-lf*Caf)/Caf/Car/(lr+lf)/2));

== matlab function DYC0928/Subsystem/Subsystem/载荷转移 ==
  data: ax input; Fz1 output; Fz2 output; Fz3 output; Fz4 output; ay input; h input; lfw input; lrw input; lf input; lr input; m input
function [Fz1,Fz2,Fz3,Fz4] = fcn(ax,ay,h,lfw,lrw,lf,lr,m)
g = 9.8;

Fz1 = (lr/(lf+lr))*(0.5*m*g-m*ay*h/lfw)-0.5*m*ax*h/(lf+lr);
Fz2 = (lr/(lf+lr))*(0.5*m*g+m*ay*h/lfw)-0.5*m*ax*h/(lf+lr);
Fz3 = (lr/(lf+lr))*(0.5*m*g-m*ay*h/lrw)+0.5*m*ax*h/(lf+lr);
Fz4 = (lr/(lf+lr))*(0.5*m*g+m*ay*h/lrw)+0.5*m*ax*h/(lf+lr);
